simulink model "KalashErrorCalculation"  (R2017a)
settings: Solver=FixedStepAuto  StartTime=0.0  StopTime=inf  RelTol=1e-3  EnableMultiTasking=on
libraries: arduinolib x8
settings Model: SimulationMode=external  ExtModeTrigDuration=2  Creator=Rutvik  LastModifiedBy=hp
settings OptimizationCC: PassReuseOutputArgsAs=Individual arguments  MaxStackSize=64
settings DebuggingCC: ParameterTunabilityLossMsg=error
settings HardwareCC: ProdBitPerInt=16  ProdBitPerPointer=16  ProdBitPerSizeT=16  ProdBitPerPtrDiffT=16  ProdLargestAtomicFloat=None  ProdWordSize=8  ProdHWDeviceType=Atmel->AVR
settings SFSimCC: MATLABDynamicMemAlloc=off
settings RTWCC: SystemTargetFile=ert.tlc  HardwareBoard=Arduino Mega 2560  TLCOptions=-aInlineSetEventsForThisBaseRateFcn=TLC_FALSE -aSuppressMultiTaskScheduler=TLC_FALSE -aRateBasedStepFcn=1  TemplateMakefile=ert_default_tmf  Description=Embedded Coder  GenerateReport=on  Toolchain=Arduino AVR  BuildConfiguration=Faster Runs  IncludeHyperlinkInReport=on  LaunchReport=on  GenerateTraceInfo=on  GenerateTraceReport=on  GenerateTraceReportSl=on  GenerateTraceReportSf=on  GenerateTraceReportEml=on
settings CodeAppCC: ForceParamTrailComments=on  IgnoreCustomStorageClasses=off  OperatorAnnotations=on  SimulinkDataObjDesc=on  SFDataObjDesc=on  MATLABFcnDesc=on  InsertBlockDesc=on  MATLABSourceComments=on
settings ERTTargetCC: SupportContinuousTime=on  SupportVariableSizeSignals=on

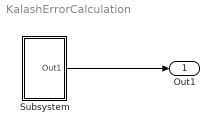
== system KalashErrorCalculation ==
  Subsystem : Subsystem
  Out1 : Outport
  wires:
  Subsystem/1(Out1) -> Out1/1

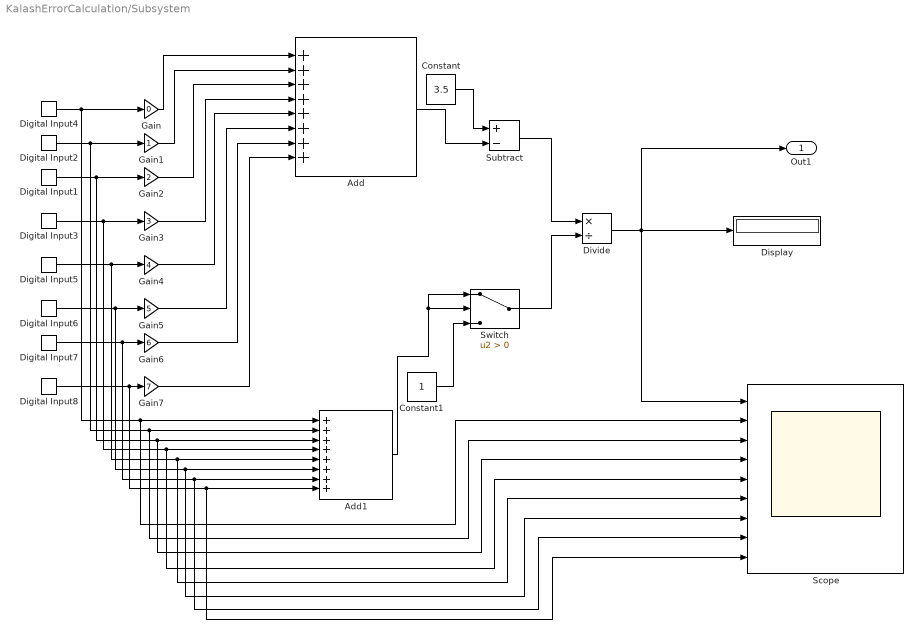
== system KalashErrorCalculation/Subsystem ==
  Add : Sum  Inputs=++++++++
  Add1 : Sum  Inputs=++++++++
  Constant : Constant  Value=3.5
  Constant1 : Constant
  Digital Input1 : arduinolib/Digital Input  pinNumber=3  sampleTime=0.002  blockPlatform=arduino
      settings: SourceProductName=Simulink Support Package for Arduino Hardware
  Digital Input2 : arduinolib/Digital Input  pinNumber=2  sampleTime=0.002  blockPlatform=arduino
      settings: SourceProductName=Simulink Support Package for Arduino Hardware
  Digital Input3 : arduinolib/Digital Input  pinNumber=4  sampleTime=0.002  blockPlatform=arduino
      settings: SourceProductName=Simulink Support Package for Arduino Hardware
  Digital Input4 : arduinolib/Digital Input  pinNumber=9  sampleTime=0.002  blockPlatform=arduino
      settings: SourceProductName=Simulink Support Package for Arduino Hardware
  Digital Input5 : arduinolib/Digital Input  pinNumber=5  sampleTime=0.002  blockPlatform=arduino
      settings: SourceProductName=Simulink Support Package for Arduino Hardware
  Digital Input6 : arduinolib/Digital Input  pinNumber=6  sampleTime=0.002  blockPlatform=arduino
      settings: SourceProductName=Simulink Support Package for Arduino Hardware
  Digital Input7 : arduinolib/Digital Input  pinNumber=7  sampleTime=0.002  blockPlatform=arduino
      settings: SourceProductName=Simulink Support Package for Arduino Hardware
  Digital Input8 : arduinolib/Digital Input  pinNumber=8  sampleTime=0.002  blockPlatform=arduino
      settings: SourceProductName=Simulink Support Package for Arduino Hardware
  Display : Display
  Divide : Product  Inputs=*/
  Gain : Gain  Gain=0
  Gain1 : Gain
  Gain2 : Gain  Gain=2
  Gain3 : Gain  Gain=3
  Gain4 : Gain  Gain=4
  Gain5 : Gain  Gain=5
  Gain6 : Gain  Gain=6
  Gain7 : Gain  Gain=7
  Scope : Scope  NumInputPorts=9
  Subtract : Sum  Inputs=+-
  Switch : Switch  Criteria=u2 > Threshold
  Out1 : Outport
  wires:
  Digital Input2/1 -> Scope/3, Add1/2, Gain1/1
  Digital Input7/1 -> Scope/8, Add1/7, Gain6/1
  Digital Input3/1 -> Scope/5, Add1/4, Gain3/1
  Add/1 -> Subtract/2
  Constant/1 -> Subtract/1
  Digital Input6/1 -> Scope/7, Add1/6, Gain5/1
  Digital Input4/1 -> Scope/2, Add1/1, Gain/1
  Switch/1 -> Divide/2
  Divide/1 -> Out1/1, Scope/1, Display/1
  Constant1/1 -> Switch/3
  Add1/1 -> Switch/1, Switch/2
  Digital Input8/1 -> Scope/9, Add1/8, Gain7/1
  Digital Input1/1 -> Scope/4, Add1/3, Gain2/1
  Subtract/1 -> Divide/1
  Digital Input5/1 -> Scope/6, Add1/5, Gain4/1
  Gain3/1 -> Add/4
  Gain1/1 -> Add/2
  Gain2/1 -> Add/3
  Gain7/1 -> Add/8
  Gain/1 -> Add/1
  Gain4/1 -> Add/5
  Gain6/1 -> Add/7
  Gain5/1 -> Add/6
